simulink model "simulation"  (R2022b)
settings: Solver=VariableStepAuto  StartTime=0.0  StopTime=18  RelTol=1e-3
values from neighbouring files (symbols this model uses):
  Abar = [Ap zeros(np,m); Cp zeros(m,m)]    [main.m]
  Adaptive_OFF = input(['\nChoose: \n'      '0: Adaptive_ON \n'      '1: Adaptive_OFF \n'      'Adaptive Type: '])    [main.m]
  B = [Bp; zeros(m,m)]    [main.m]
  Bc = [zeros(np,m); -eye(m)]    [main.m]
  C = [Cp zeros(m,m)]    [main.m]
  Gamma = eye(p)*gamma    [main.m]
  Kbl = -K    [main.m]
  Lambda = eye(m)    [main.m]
  P = lyap(Am.',eye(n))    [main.m]
  quad = droneParams    [main.m]    (also in provaMatrici.m)
  simulationType = input(['Choose simulation type: \n'      '1: Regulation \n'      '2: RegulationMultiple \n'      '3: Tracking \n'      'Simulation Type: '])    [main.m]
  t_failure = 60    [main.m]
settings Model: Creator=aleix  LastModifiedBy=Musta
settings SolverCC: AlgebraicLoopSolver=TrustRegion
settings DebuggingCC: UnconnectedInputMsg=warning  UnconnectedOutputMsg=warning  UnconnectedLineMsg=warning  SFMachineParentedDataDiag=warning
settings ModelReferenceCC: EnableRefExpFcnMdlSchedulingChecks=on

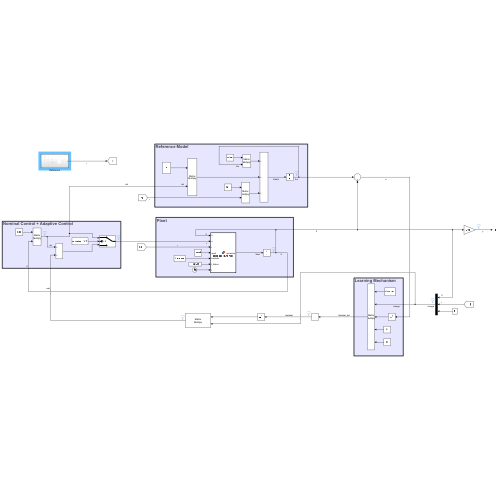
[thumbnail: Simulink's stored preview of the top-level diagram]
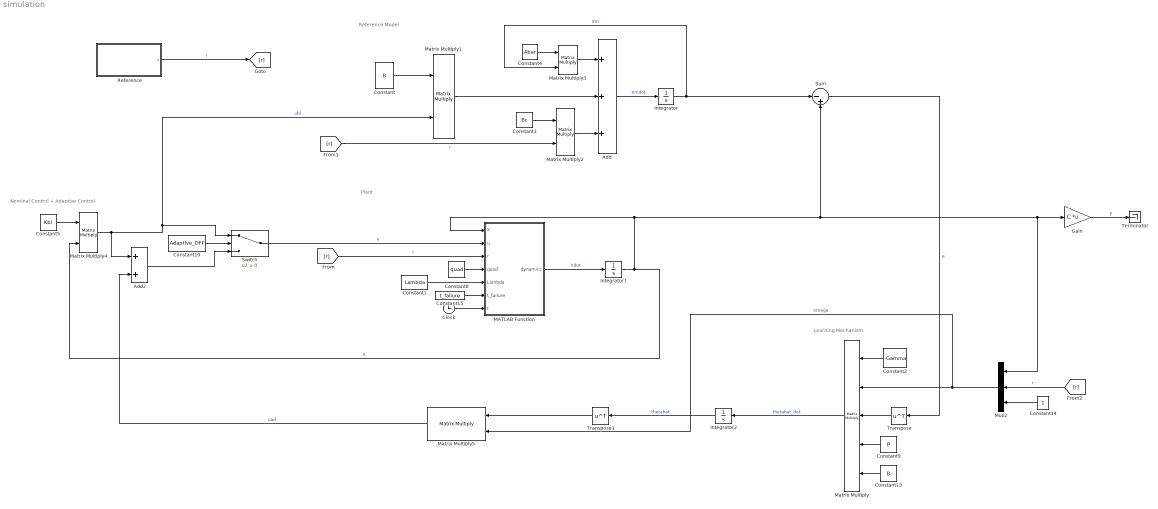
== system simulation ==
  note: Learning Mechanism
  note: Nominal Control + Adaptive Control
  note: Plant
  note: Reference Model
  Add : Sum  Inputs=3
  Add2 : Sum
  Clock : Clock
  Constant : Constant  Value=B
  Constant1 : Constant  Value=Lambda
  Constant10 : Constant  Value=Adaptive_OFF
  Constant13 : Constant  Value=B
  Constant14 : Constant  VectorParams1D=off
  Constant15 : Constant  Value=t_failure
  Constant2 : Constant  Value=-Gamma
  Constant3 : Constant  Value=Bc
  Constant4 : Constant  Value=Abar
  Constant5 : Constant  Value=Kbl
  Constant8 : Constant  Value=quad  OutDataTypeStr=Bus: slBus1
  Constant9 : Constant  Value=P
  Gain : Gain  Gain=C  Multiplication=Matrix(K*u)
  Integrator : Integrator
  Integrator1 : Integrator
  Integrator2 : Integrator
  MATLAB Function : MATLAB Function  TreatAsAtomicUnit=on
  Matrix Multiply : Product  Inputs=5  Multiplication=Matrix(*)
  Matrix Multiply{1..5} (5 alike) : Product  Multiplication=Matrix(*)
  Mux2 : Mux  Inputs=3
  Reference : Subsystem
  Sum : Sum  Inputs=|-+
  Switch : Switch  Criteria=u2 > Threshold  SaturateOnIntegerOverflow=off  InputSameDT=off
  Terminator : Terminator
  Transpose : Math  Operator=transpose
  Transpose1 : Math  Operator=transpose
  wires:
  [r] -> Mux2/2  "r"
  Mux2/1 -> Matrix Multiply5/2, Matrix Multiply/2  "omega"
  Transpose/1 -> Matrix Multiply/3
  Matrix Multiply5/1 -> Add2/2  "uad"
  [r] -> Matrix Multiply2/2  "r"
  Constant/1 -> Matrix Multiply1/1
  Matrix Multiply4/1 -> Add2/1, Matrix Multiply1/2, Switch/1  "ubl"
  Constant8/1 -> MATLAB Function/4(quad)
  Constant14/1 -> Mux2/3
  Matrix Multiply2/1 -> Add/3
  Constant4/1 -> Matrix Multiply3/1
  Transpose1/1 -> Matrix Multiply5/1
  Constant1/1 -> MATLAB Function/5(Lambda)
  Clock/1 -> MATLAB Function/7(t)
  Constant15/1 -> MATLAB Function/6(t_failure)
  [r] -> MATLAB Function/3(r)  "r"
  Constant13/1 -> Matrix Multiply/5
  Switch/1 -> MATLAB Function/2(u)  "u"
  Constant5/1 -> Matrix Multiply4/1
  Constant3/1 -> Matrix Multiply2/1
  Integrator1/1 -> Matrix Multiply4/2, Sum/2, Mux2/1, Gain/1, MATLAB Function/1(X)  "X"
  MATLAB Function/1(dynamics) -> Integrator1/1  "Xdot"
  Matrix Multiply/1 -> Integrator2/1  "thetahat_dot"
  Add2/1 -> Switch/3
  Matrix Multiply3/1 -> Add/1
  Integrator2/1 -> Transpose1/1  "thetahat"
  Constant9/1 -> Matrix Multiply/4
  Integrator/1 -> Matrix Multiply3/2, Sum/1  "Xm"
  Sum/1 -> Transpose/1  "e"
  Matrix Multiply1/1 -> Add/2
  Constant2/1 -> Matrix Multiply/1
  Add/1 -> Integrator/1  "Xmdot"
  Constant10/1 -> Switch/2
  Gain/1 -> Terminator/1  "y"
  Reference/1(r) -> [r]  "r"

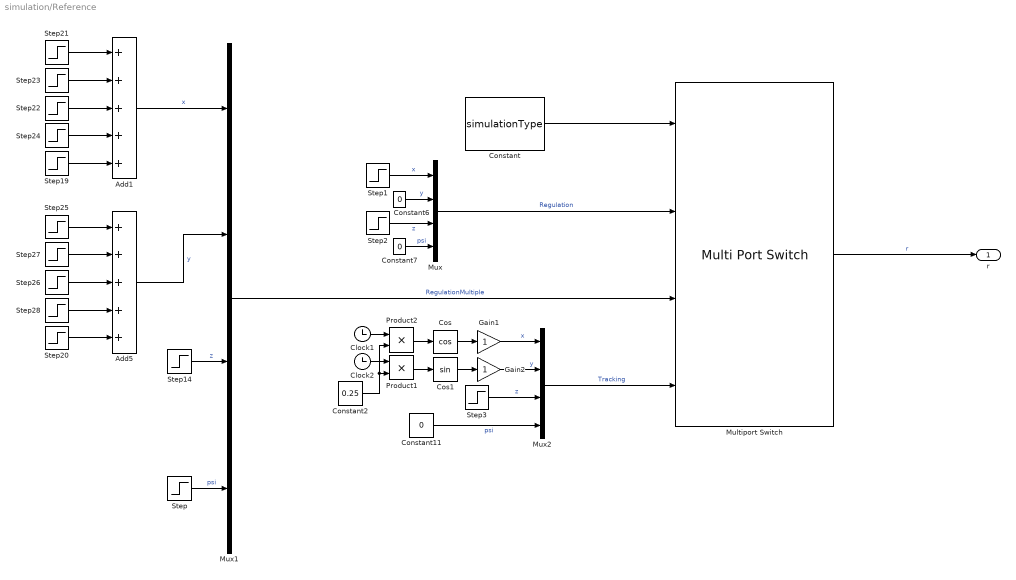
== system simulation/Reference ==
  Add1 : Sum  Inputs=+++++
  Add5 : Sum  Inputs=+++++
  Clock1 : Clock
  Clock2 : Clock
  Constant : Constant  Value=simulationType
  Constant11 : Constant  Value=0
  Constant2 : Constant  Value=0.25
  Constant6 : Constant  Value=0
  Constant7 : Constant  Value=0
  Cos : Trigonometry  Operator=cos
  Cos1 : Trigonometry
  Gain1 : Gain
  Gain2 : Gain
  Multiport Switch : MultiPortSwitch  SaturateOnIntegerOverflow=off  InputSameDT=off
  Mux : Mux
  Mux1 : Mux
  Mux2 : Mux
  Product1 : Product
  Product2 : Product
  Step : Step  Time=0  After=0  SampleTime=0
  Step1 : Step  SampleTime=0
  Step14 : Step  After=5  SampleTime=0
  Step19 : Step  Time=50  After=2  SampleTime=0
  Step2 : Step  After=5  SampleTime=0
  Step20 : Step  Time=50  After=0  SampleTime=0
  Step21 : Step  Time=10  SampleTime=0
  Step22 : Step  Time=30  After=-2  SampleTime=0
  Step23 : Step  Time=20  After=0  SampleTime=0
  Step24 : Step  Time=40  After=0  SampleTime=0
  Step25 : Step  Time=10  After=-1  SampleTime=0
  Step26 : Step  Time=30  After=0  SampleTime=0
  Step27 : Step  Time=20  After=2  SampleTime=0
  Step28 : Step  Time=40  After=-2  SampleTime=0
  Step3 : Step  Time=0  After=5  SampleTime=0
  r : Outport
  wires:
  Step27/1 -> Add5/2
  Step24/1 -> Add1/4
  Step28/1 -> Add5/4
  Step26/1 -> Add5/3
  Step22/1 -> Add1/3
  Step25/1 -> Add5/1
  Step23/1 -> Add1/2
  Step21/1 -> Add1/1
  Step20/1 -> Add5/5
  Add1/1 -> Mux1/1  "x"
  Step19/1 -> Add1/5
  Mux1/1 -> Multiport Switch/3  "RegulationMultiple"
  Add5/1 -> Mux1/2  "y"
  Step14/1 -> Mux1/3  "z"
  Step/1 -> Mux1/4  "psi"
  Multiport Switch/1 -> r/1  "r"
  Constant7/1 -> Mux/4  "psi"
  Step2/1 -> Mux/3  "z"
  Step1/1 -> Mux/1  "x"
  Mux/1 -> Multiport Switch/2  "Regulation"
  Constant6/1 -> Mux/2  "y"
  Clock1/1 -> Product2/1
  Constant11/1 -> Mux2/4  "psi"
  Constant2/1 -> Product2/2, Product1/2
  Gain2/1 -> Mux2/2  "y"
  Cos1/1 -> Gain2/1
  Cos/1 -> Gain1/1
  Clock2/1 -> Product1/1
  Product1/1 -> Cos1/1
  Gain1/1 -> Mux2/1  "x"
  Mux2/1 -> Multiport Switch/4  "Tracking"
  Step3/1 -> Mux2/3  "z"
  Product2/1 -> Cos/1
  Constant/1 -> Multiport Switch/1

== matlab function simulation/MATLAB Function ==
  data: X input size=[16 1]; dynamics output size=[16 1]; u input size=[4 1]; r input size=[4 1]; quad input; Lambda input; t_failure input; t input
function dynamics = compute_dynamics(X, u, r, quad, Lambda, t_failure, t)

dynamics = zeros(16,1);

% Datas
g  = quad.g;
m  = quad.M;
Ix = quad.Ix;
Iy = quad.Iy;
Iz = quad.Iz;
L  = quad.d;
Jr = quad.Ir;
omegar = quad.omegar;

% Dynamics
pos_x                  = X(1);
pos_y                  = X(2);
pos_z                  = X(3);
phi                    = X(4);
theta                  = X(5);
psi                    = X(6);
vel_x                  = X(7);
vel_y                  = X(8);
vel_z                  = X(9);
phi_dot                = X(10);
theta_dot              = X(11);
psi_dot                = X(12);
% eyI not used

if t < t_failure  % no failure before t_faliure
    Lambda = eye(size(Lambda));
end

% TODO: impose actuator saturation
U = [m*g + u(1); u(2); u(3); u(4)]; % u(1) is deltaU1
U_fail = quad.H*Lambda*quad.H_inv*U;
U1 = U_fail(1);
U2 = U_fail(2);
U3 = U_fail(3);
U4 = U_fail(4);

sphi   = sin(phi);
stheta = sin(theta);
spsi   = sin(psi);
cphi   = cos(phi);
ctheta = cos(theta);
cpsi   = cos(psi);
%ttheta = tan(theta);

pos_dot_x     = vel_x;
pos_dot_y     = vel_y;
pos_dot_z     = vel_z;
orient_dot_x  = phi_dot;  % p + r.*(cphi.*ttheta) + q.*(sphi.*ttheta);
orient_dot_y  = theta_dot;  % q.*cphi - r.*sphi;
orient_dot_z  = psi_dot;  % r.*cphi./ctheta + q.*sphi./ctheta;

vel_dot_x     = U1.*(sphi.*spsi + cphi.*cpsi.*stheta)./m; %- Axyz(1).*vel_x./m;
vel_dot_y     = U1.*(cphi.*spsi.*stheta - cpsi.*sphi)./m; %- Axyz(2).*vel_y./m;
vel_dot_z     = U1.*(cphi.*ctheta)./m - g;                %- Axyz(3).*vel_z./m;

rate_dot_x    = ((Iy - Iz).*psi_dot.*theta_dot - Jr.*theta_dot.*omegar + L.*U2)./Ix;
rate_dot_y    = ((Iz - Ix).*phi_dot.*psi_dot + Jr.*phi_dot.*omegar + L.*U3)./Iy;
rate_dot_z    = ((Ix - Iy).*phi_dot.*theta_dot + U4)./Iz;

eyIx_dot = pos_x - r(1);
eyIy_dot = pos_y - r(2);
eyIz_dot = pos_z - r(3);
eyIpsi_dot = psi - r(4);

dynamics = [
    pos_dot_x; pos_dot_y; pos_dot_z; ...
    orient_dot_x; orient_dot_y; orient_dot_z; 
    vel_dot_x; vel_dot_y; vel_dot_z;  ...
    rate_dot_x; rate_dot_y; rate_dot_z; 
    eyIx_dot; eyIy_dot; eyIz_dot; eyIpsi_dot ...
];

end
